simulink model "BERS"  (R2020a)
settings: Solver=VariableStepAuto  StartTime=0.0  StopTime=10.0  RelTol=1e-3
model workspace (MAT data in the model file):
  Batt.init_charge = 100
  Batt.Vnom = 320
  Batt.Ah_rating = 100
  Batt.R1 = 0.0846
  Batt.V1 = 283.3
  Batt.Q1 = 10.4
  Batt.Limit.SOC = [0 10 20 30 40 50 60 70 80 90 100]
  Batt.Limit.Discharge = [0 15000 33000 54000 75000 90000 108000 117000 120000 120000 120000]
  Batt.Limit.Charge = [1 1 1 1 1 1 1 1 0.75 0.35 0]
  Batt.m = 119.7
  Batt.Cp = 101.079756
libraries: simulink x1
settings Model: Creator=Administrator  LastModifiedBy=Administrator

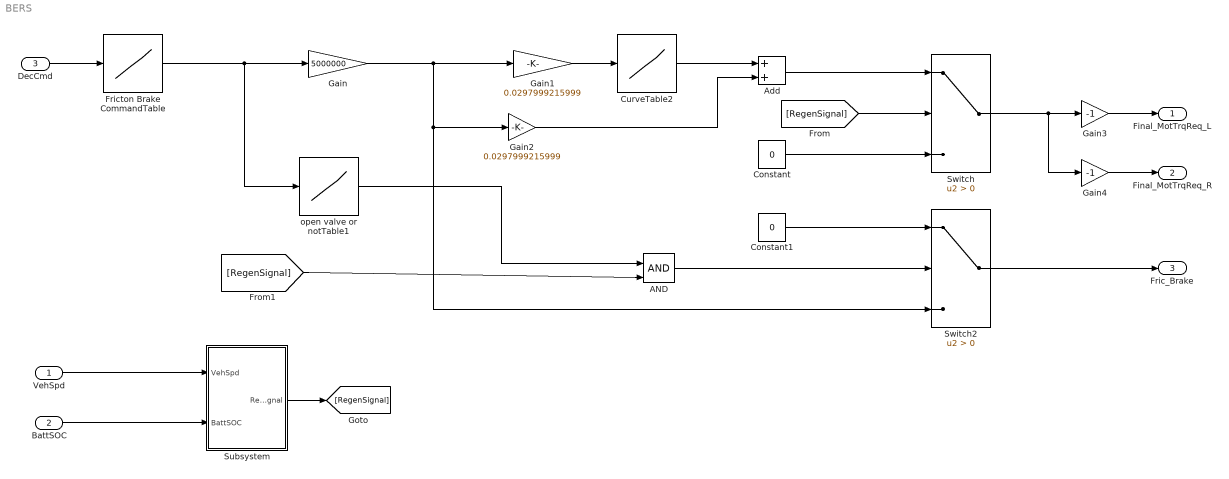
== system BERS ==
  VehSpd : Inport
  BattSOC : Inport  Port=2
  DecCmd : Inport  Port=3
  AND : Logic  IconShape=distinctive  AllPortsSameDT=off  OutDataTypeStr=boolean
  Add : Sum
  Constant : Constant  Value=0
  Constant1 : Constant  Value=0
  CurveTable2 : Lookup_n-D  NumberOfTableDimensions=1  BreakpointsForDimension1=Batt.Limit.SOC  Table=Batt.Limit.Charge  InternalRulePriority=Speed  RndMeth=Simplest  InputSameDT=on
  Fricton Brake CommandTable : Lookup_n-D  NumberOfTableDimensions=1  BreakpointsForDimension1=[.0 0.1 0.2 0.4 0.6 0.8 1.0]  Table=[0 0 0.2 0.4 0.6 0.8 1.0]*60  InternalRulePriority=Speed  RndMeth=Simplest  InputSameDT=on
  Gain : Gain  Gain=5000000
  Gain1 : Gain  Gain=0.0297999215999
  Gain2 : Gain  Gain=0.0297999215999
  Gain3 : Gain  Gain=-1
  Gain4 : Gain  Gain=-1
  Subsystem : Subsystem
  Switch : Switch  Criteria=u2 > Threshold
  Switch2 : Switch  Criteria=u2 > Threshold
  open valve or notTable1 : Lookup_n-D  NumberOfTableDimensions=1  BreakpointsForDimension1=[.0 0.1 0.2 0.4 0.6 0.8 1.0]  Table=[0 0 0.2 0.4 0.6 0.8 1.0]*60  InternalRulePriority=Speed  RndMeth=Simplest  InputSameDT=on
  Final_MotTrqReq_L : Outport
  Final_MotTrqReq_R : Outport  Port=2
  Fric_Brake : Outport  Port=3
  wires:
  DecCmd/1 -> Fricton Brake CommandTable/1
  Fricton Brake CommandTable/1 -> open valve or notTable1/1, Gain/1
  Gain/1 -> Switch2/3, Gain2/1, Gain1/1
  Gain1/1 -> CurveTable2/1
  CurveTable2/1 -> Add/1
  Gain2/1 -> Add/2
  open valve or notTable1/1 -> AND/1
  Add/1 -> Switch/1
  Constant/1 -> Switch/3
  [RegenSignal] -> Switch/2
  [RegenSignal] -> AND/2
  AND/1 -> Switch2/2
  Constant1/1 -> Switch2/1
  Switch/1 -> Gain4/1, Gain3/1
  Gain3/1 -> Final_MotTrqReq_L/1
  Gain4/1 -> Final_MotTrqReq_R/1
  Switch2/1 -> Fric_Brake/1
  VehSpd/1 -> Subsystem/1(VehSpd)
  BattSOC/1 -> Subsystem/2(BattSOC)
  Subsystem/1(RegenSignal) -> [RegenSignal]

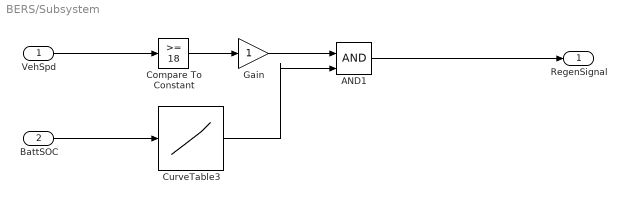
== system BERS/Subsystem ==
  VehSpd : Inport
  BattSOC : Inport  Port=2
  AND1 : Logic  IconShape=distinctive  AllPortsSameDT=off  OutDataTypeStr=boolean
  Compare To Constant : simulink/Logic and Bit Operations/Compare To Constant  relop=>=  const=18  OutDataTypeStr=boolean
  CurveTable3 : Lookup_n-D  NumberOfTableDimensions=1  BreakpointsForDimension1=Batt.Limit.SOC  Table=Batt.Limit.Charge  InternalRulePriority=Speed  RndMeth=Simplest  InputSameDT=on
  Gain : Gain
  RegenSignal : Outport
  wires:
  VehSpd/1 -> Compare To Constant/1
  CurveTable3/1 -> AND1/2
  BattSOC/1 -> CurveTable3/1
  AND1/1 -> RegenSignal/1
  Gain/1 -> AND1/1
  Compare To Constant/1 -> Gain/1
